simulink model "actuation"  (R2019b)
settings: Solver=ode45  StartTime=0.0  StopTime=5  RelTol=1e-3  EnableMultiTasking=on
undefined symbols (not defined in the file or in its folder): DiscIntNeverNeededParam
libraries: truetime x4, visionstatistics x1
settings Model: Creator=anton  LastModifiedBy=carlosxavierroserochandi
settings DataIOCC: LimitDataPoints=on  SaveFormat=Array  ReturnWorkspaceOutputs=off
settings OptimizationCC: ExpressionDepthLimit=2147483647  LifeSpan=inf
settings DebuggingCC: UnderspecifiedInitializationDetection=Classic  MergeDetectMultiDrivingBlocksExec=none  FcnCallInpInsideContextMsg=warning  StateNameClashWarn=warning  SFUnexpectedBacktrackingDiag=warning  SFNoUnconditionalDefaultTransitionDiag=warning  SFExecutionAtInitializationDiag=none  ArithmeticOperatorsInVariantConditions=warning
settings HardwareCC: ProdBitPerPointer=32  ProdBitPerSizeT=32  ProdBitPerPtrDiffT=32  ProdLargestAtomicFloat=None  ProdIntDivRoundTo=Undefined  ProdEndianess=Unspecified  ProdWordSize=32  ProdHWDeviceType=32-bit Generic
settings ModelReferenceCC: PropagateSignalLabelsOutOfModel=off
settings SFSimCC: SimUseLocalCustomCode=off  CustomCodeUndefinedFunction=UseInterfaceOnly
settings RTWCC: RTWUseLocalCustomCode=off
settings CodeAppCC: StateflowObjectComments=on
settings GRTTargetCC: TargetLangStandard=C89/C90 (ANSI)  GeneratePreprocessorConditionals=Disable all
settings ConfigComp: CovMetricSettings=dw  CovHtmlReporting=on  CovSaveCumulativeToWorkspaceVar=on  CovSaveSingleToWorkspaceVar=on  CovExternalEMLEnable=off

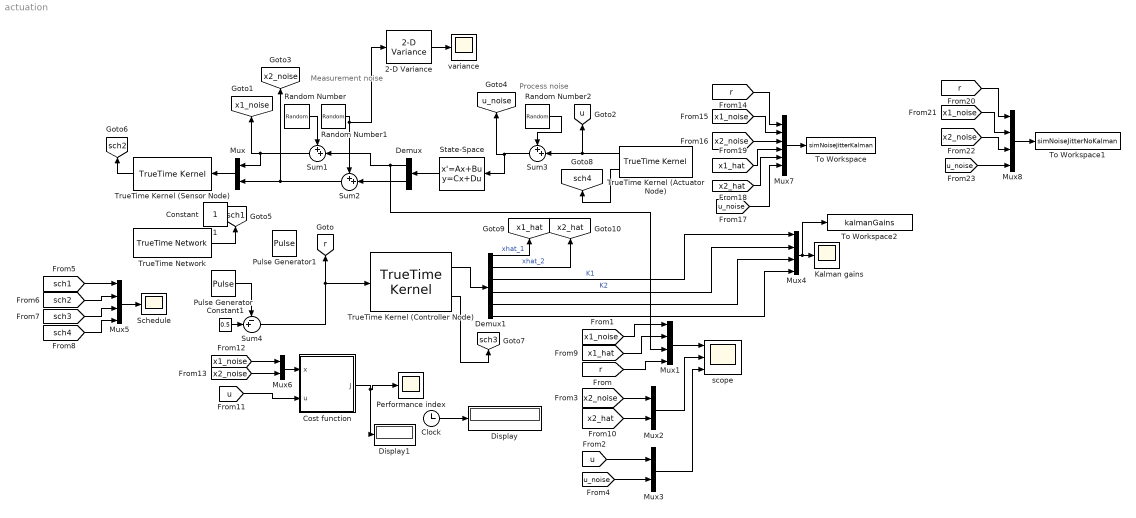
== system actuation ==
  note: Process
      | noise
  note: Measurement
      | noise
  2-D Variance : visionstatistics/2-D Variance  run=on  reset_popup=None  directionMode=Specified dimension  dimension=1  treatSBRowAsCol=on  roiEnable=off  roiType=Rectangles  roiPortion=ROI perimeter  roiOutput=Individual statistics for each ROI  roiFlag=off  roundingMode=Floor  overflowMode=off  prodOutputMode=Binary point scaling  prodOutputWordLength=32  prodOutputFracLength=0  prodOutputSlope=2^0  memorySlope=2^-30  accumSlope=2^-32  outputSlope=2^-32
      settings: SourceProductName=Computer Vision Toolbox  SourceProductBaseCode=VP
  Clock : Clock
  Constant1 : Constant  Value=0.5
  Cost function : Subsystem
  Demux : Demux  Outputs=2
  Demux1 : Demux  Outputs=6
  Display : Display
  Display1 : Display
  Kalman gains : Scope
  Mux{,2..3,6} (4 alike) : Mux  Inputs=2
  Mux{1,4..5,8} (4 alike) : Mux
  Mux7 : Mux  Inputs=6
  Performance index : Scope
  Pulse Generator : DiscretePulseGenerator  PulseType=Time based  Period=5  PulseWidth=50  PhaseDelay=0.01
  Pulse Generator1 : DiscretePulseGenerator  PulseType=Time based  Amplitude=0.5  Period=5  PulseWidth=0.5
  Random Number : RandomNumber  Variance=0.001*20e-3  Seed=1534  SampleTime=0.01
  Random Number1 : RandomNumber  Variance=0.003*20e-3  Seed=109  SampleTime=0.01
  Random Number2 : RandomNumber  Variance=0.0001*20e-3  Seed=100  SampleTime=0.01
  Schedule : Scope
  State-Space : StateSpace  A=[0 -23.8095; 0 0];  B=[0; -23.8095];  C=[1 0; 0 1]  D=[0; 0]  InitialCondition=0
  Sum1 : Sum  Inputs=++|  SaturateOnIntegerOverflow=on  InputSameDT=on  OutDataTypeStr=Inherit: Same as first input
  Sum2 : Sum  Inputs=++|  SaturateOnIntegerOverflow=on  InputSameDT=on  OutDataTypeStr=Inherit: Same as first input
  Sum3 : Sum  Inputs=++|  SaturateOnIntegerOverflow=on  InputSameDT=on  OutDataTypeStr=Inherit: Same as first input
  Sum4 : Sum  Inputs=-+|  SaturateOnIntegerOverflow=on  InputSameDT=on  OutDataTypeStr=Inherit: Same as first input
  To Workspace : ToWorkspace  VariableName=simNoiseJitterKalman  SaveFormat=Structure With Time  SampleTime=-1
  To Workspace1 : ToWorkspace  VariableName=simNoiseJitterNoKalman  SaveFormat=Structure With Time  SampleTime=-1
  To Workspace2 : ToWorkspace  VariableName=kalmanGains  SaveFormat=Structure With Time  SampleTime=-1
  TrueTime Kernel (Actuator Node) : truetime/TrueTime Kernel  sfun=actuator_init  args=[]  ninputsoutputs=[0 1]  ntriggers=0  trigtype=rising  nwnodenbr=4  clockoffsetdrift=[0 0]  schedoutput=on  battery=off  poweroutput=off  label=1: 4
  TrueTime Kernel (Controller Node) : truetime/TrueTime Kernel  sfun=controller_init  args=0.0  ninputsoutputs=[1 6]  ntriggers=0  trigtype=rising  nwnodenbr=3  clockoffsetdrift=[0 0]  schedoutput=on  battery=off  poweroutput=off  label=1: 3
  TrueTime Kernel (Sensor Node) : truetime/TrueTime Kernel  sfun=sensor_init  args=[]  ninputsoutputs=[2 0]  ntriggers=0  trigtype=rising  nwnodenbr=2  clockoffsetdrift=[0 0]  schedoutput=on  battery=off  poweroutput=off  label=1: 2
  "TrueTime Network " : truetime/TrueTime Network  nwtype=CSMA/CD (Ethernet)  nwnbr=1  nnodes=4  rate=80000  minsize=80  lossprob=0  seed=0  bandwidths=[0.5 0.25 0.25]  slotsize=80  schedule=[1 2 1 3]  memsize=80000  buftype=Common buffer  overflow=Retransmit  dynSchedule=[]  miniSlotSize=40  NIT=0  QSortMode=FIFO  sync=0  irtSchedule=0  nrtLength=0  nodeGraph=0  scheduleoutput=on
  scope : Scope  NumInputPorts=3
  variance : Scope
  1 : Constant  IOType=siggen
  Constant : Constant  IOType=siggen
  tag scope: r=global, sch1=global, sch2=global, sch3=global, sch4=global, u=global, u_noise=global, x1_hat=global, x1_noise=global, x2_hat=global, x2_noise=global
  wires:
  Mux1/1 -> scope/1
  Clock/1 -> Display/1
  State-Space/1 -> Demux/1
  Demux/1 -> Mux1/3, Sum1/2
  Demux/2 -> Sum2/2
  Sum1/1 -> Mux/1, [x1_noise]
  Sum2/1 -> [x2_noise], Mux/2
  Sum3/1 -> [u_noise], State-Space/1
  TrueTime Kernel (Actuator Node)/1 -> [u], Sum3/2
  TrueTime Kernel (Controller Node)/1 -> Demux1/1
  [x2_noise] -> Mux2/1
  Demux1/2 -> [x2_hat]  "xhat_2"
  Mux2/1 -> scope/2
  [u] -> Mux3/1
  [u_noise] -> Mux3/2
  Mux3/1 -> scope/3
  [x1_noise] -> Mux1/1
  Demux1/3 -> Mux4/1  "K1"
  Mux4/1 -> To Workspace2/1, Kalman gains/1
  Demux1/4 -> Mux4/2  "K2"
  Mux5/1 -> Schedule/1
  Random Number1/1 -> Sum2/1, 2-D Variance/1
  "TrueTime Network "/1 -> [sch1]
  TrueTime Kernel (Sensor Node)/1 -> [sch2]
  TrueTime Kernel (Controller Node)/2 -> [sch3]
  TrueTime Kernel (Actuator Node)/2 -> [sch4]
  [sch1] -> Mux5/1
  [sch2] -> Mux5/2
  [sch3] -> Mux5/3
  [sch4] -> Mux5/4
  Demux1/1 -> [x1_hat]  "xhat_1"
  [x1_hat] -> Mux1/2
  [x2_hat] -> Mux2/2
  Pulse Generator/1 -> Sum4/1
  2-D Variance/1 -> variance/1
  [r] -> Mux1/4
  Mux/1 -> TrueTime Kernel (Sensor Node)/1
  Cost function/1(J) -> Display1/1, Performance index/1
  [u] -> Cost function/2(u)
  [x1_noise] -> Mux6/1
  [x2_noise] -> Mux6/2
  Mux6/1 -> Cost function/1(x)
  Demux1/5 -> Mux4/3
  Demux1/6 -> Mux4/4
  Mux7/1 -> To Workspace/1
  [r] -> Mux7/1
  [x1_noise] -> Mux7/2
  [x2_noise] -> Mux7/3
  Constant1/1 -> Sum4/2
  [x1_hat] -> Mux7/4
  [x2_hat] -> Mux7/5
  [u_noise] -> Mux7/6
  [r] -> Mux8/1
  [x1_noise] -> Mux8/2
  Mux8/1 -> To Workspace1/1
  [x2_noise] -> Mux8/3
  [u_noise] -> Mux8/4
  Random Number/1 -> Sum1/1
  Random Number2/1 -> Sum3/1
  Sum4/1 -> TrueTime Kernel (Controller Node)/1, [r]

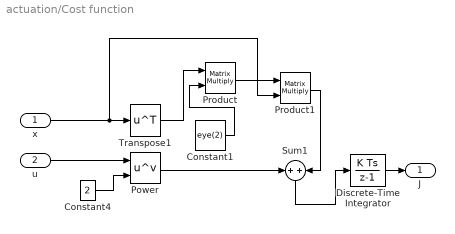
== system actuation/Cost function ==
  x : Inport
  u : Inport  Port=2
  Constant1 : Constant  Value=eye(2)  SampleTime=-1
  Constant4 : Constant  Value=2  SampleTime=-1
  Discrete-Time Integrator : DiscreteIntegrator  SampleTime=-1  ICPrevOutput=DiscIntNeverNeededParam  ICPrevScaledInput=DiscIntNeverNeededParam
  Power : Math  Operator=pow  SignedPower=off  SaturateOnIntegerOverflow=on
  Product : Product  Multiplication=Matrix(*)
  Product1 : Product  Multiplication=Matrix(*)
  Sum1 : Sum
  Transpose1 : Math  Operator=transpose  SignedPower=off  SaturateOnIntegerOverflow=on
  J : Outport
  wires:
  u/1 -> Power/1
  Constant1/1 -> Product/2
  Constant4/1 -> Power/2
  Transpose1/1 -> Product/1
  Power/1 -> Sum1/1
  Product/1 -> Product1/1
  Product1/1 -> Sum1/2
  x/1 -> Product1/2, Transpose1/1
  Discrete-Time Integrator/1 -> J/1
  Sum1/1 -> Discrete-Time Integrator/1
